simulink model "sine_product"  (R2017b)
settings: Solver=VariableStepAuto  StartTime=0.0  StopTime=0.1  RelTol=1e-3
libraries: dspsnks4 x1
settings Model: Creator=think  LastModifiedBy=think

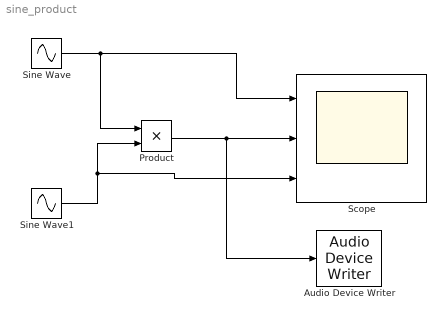
== system sine_product ==
  Audio Device Writer : dspsnks4/Audio Device Writer  Driver=DirectSound  Device=Default  InheritSampleRate=on  SampleRate=44100  BitDepth=16-bit integer  BufferSize=4096  NumBuffers=10  DefaultOutputChannelMapping=on  OutputChannelMapping=1:2  OutputNumUnderrunSamples=off  DriverIdx=1  DeviceWarnFlag=''
  Product : Product
  Scope : Scope  NumInputPorts=3
  Sine Wave : Sin  SineType=Sample based  Frequency=2*pi*31.25  Samples=1536  SampleTime=1/48000
  Sine Wave1 : Sin  SineType=Sample based  Frequency=2*pi*500  Samples=96  SampleTime=1/48000
  wires:
  Sine Wave/1 -> Product/1, Scope/1
  Sine Wave1/1 -> Product/2, Scope/3
  Product/1 -> Audio Device Writer/1, Scope/2
